simulink model "VTP"  (R2016b)
settings: Solver=VariableStepAuto  StartTime=0.0  StopTime=100.0  RelTol=1e-3
libraries: fuzblock x1
settings Model: Creator=Mohammad  LastModifiedBy=Mohammad

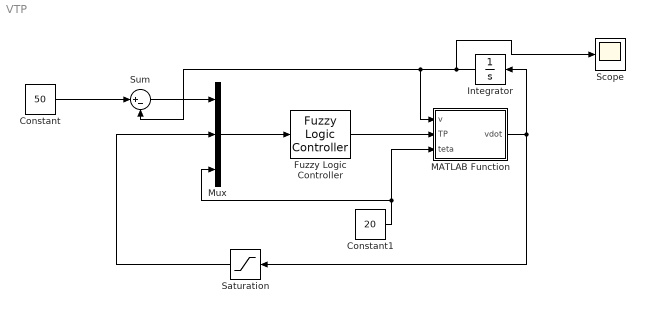
== system VTP ==
  Constant : Constant  Value=50
  Constant1 : Constant  Value=20
  Fuzzy Logic Controller : fuzblock/Fuzzy Logic  Controller  fis=Fuzzy
  Integrator : Integrator
  MATLAB Function : MATLAB Function  TreatAsAtomicUnit=on
  Mux : Mux  Inputs=3
  Saturation : Saturate
  Scope : Scope
  Sum : Sum  Inputs=|+-
  wires:
  Constant/1 -> Sum/1
  Sum/1 -> Mux/1
  MATLAB Function/1(vdot) -> Saturation/1, Integrator/1
  Saturation/1 -> Mux/2
  Mux/1 -> Fuzzy Logic Controller/1
  Fuzzy Logic Controller/1 -> MATLAB Function/2(TP)
  Constant1/1 -> MATLAB Function/3(teta), Mux/3
  Integrator/1 -> Scope/1, Sum/2, MATLAB Function/1(v)

== matlab function VTP/MATLAB Function ==
  data: v input; vdot output; TP input; teta input
function vdot = fcn(v,TP,teta)

vdot = -0.1*v+TP+0.1*teta;
